simulink model "SwPenSUSim_US1"  (R2021a)
settings: Solver=ode14x  StartTime=0.0  StopTime=100  FixedStep=0.001  MaxStep=0.001  RelTol=1e5
undefined symbols (not defined in the file or in its folder): X, Y, Z
libraries: sm_lib x15, nesl_utility x3
settings Model: Creator=User  LastModifiedBy=sujay
settings SolverCC: SolverJacobianMethodControl=FullAnalytical  ZeroCrossControl=DisableAll  AlgebraicLoopSolver=TrustRegion  SolverResetMethod=Robust
settings DataIOCC: ReturnWorkspaceOutputs=off
settings DebuggingCC: SFMachineParentedDataDiag=warning  ArithmeticOperatorsInVariantConditions=warning
settings SFSimCC: SimUseLocalCustomCode=off  CustomCodeUndefinedFunction=UseInterfaceOnly
settings RTWCC: RTWUseLocalCustomCode=off
settings CodeAppCC: StateflowObjectComments=on
settings SimscapeCC: SimscapeNormalizeSystem=off
settings ExplorerConfigSet: InternalSimMechanicsExplorerSettings="<ExplorerConfiguration><canonicalview>default</canonicalview><AnimationSetting><BasePlaybackSpeed>1.0</BasePlaybackSpeed><PlaybackSpeedFactor>1.0</PlaybackSpeedFactor></AnimationSetting><TilePanel><TileInfo><Tiles Columns=\"2\" Count=\"4\" Rows=\"2\"><Column Weight=\"0.4995\"/><Column Weight=\"0.5005\"/><Row Weight=\"0.5\"/><Row Weight=\"0.5\"/><Tile Height=\"1\" Width=\"1\" X=\"0\" Y=\"0\"/><Tile Height=\"1\" Width=\"1\" X=\"0\" Y=\"1\"/><Tile Height=\"1\" Width=\"1\" X=\"1\" Y=\"0\"/><Tile Height=\"1\" Width=\"1\" X=\"1\" Y=\"1\"/></Tiles></TileInfo><SceneInfo><SceneViewer><BGColor><R>0.60000002384185791</R><G>0.60000002384185791</G><B>0.60000002384185791</B></BGColor><Camera><DoPerspective>off</DoPerspective><Position><X>-0.0531052448703034363</X><Y>-1</Y><Z>-0.0866656671353977226</Z></Position><Center><X>-0.0531052448703034363</X><Y>1.38777878078144568e-17</Y><Z>-0.0866656671353977226</Z></Center><Up><X>0</X><Y>-0</Y><Z>1</Z></Up><ViewLimDist>1</ViewLimDist><YLim>0.890956787716308041</YLim><XLim>1.8773732312593634</XLim></Camera></SceneViewer><SceneViewer><BGColor><R>0.60000002384185791</R><G>0.60000002384185791</G><B>0.60000002384185791</B></BGColor><Camera><DoPerspective>off</DoPerspective><Position><X>-0.0296964864584461918</X><Y>-0.0267970504804747045</Y><Z>0.876248933374882633</Z></Position><Center><X>-0.0296964864584461918</X><Y>-0.0267970504804747045</Y><Z>-0.123751066625117367</Z></Center><Up><X>0</X><Y>1</Y><Z>-0</Z></Up><ViewLimDist>1</ViewLimDist><YLim>0.835585083440608556</YLim><XLim>1.76069714010699663</XLim></Camera></SceneViewer><SceneViewer><BGColor><R>0.60000002384185791</R><G>0.60000002384185791</G><B>0.60000002384185791</B></BGColor><Camera><DoPerspective>off</DoPerspective><Position><X>1</X><Y>-0.0387358476867863816</Y><Z>-0.0757430226595436767</Z></Position><Center><X>0</X><Y>-0.0387358476867863816</Y><Z>-0.0757430226595436767</Z></Center><Up><X>-0</X><Y>0</Y><Z>1</Z></Up><ViewLimDist>1</ViewLimDist><YLim>0.674834154997757341</YLim><XLim>1.42347829569839446</XLim></Camera></SceneViewer><SceneViewer><BGColor><R>0.60000002384185791</R><G>0.60000002384185791</G><B>0.60000002384185791</B></BGColor><Camera><DoPerspective>off</DoPerspective><Position><X>0.534397979001275503</X><Y>-0.548841185035268575</Y><Z>0.55129295382820287</Z></Position><Center><X>-0.0429522901883504296</X><Y>0.0285090841543572567</Y><Z>-0.0260573153614229794</Z></Center><Up><X>-0.408248290463863073</X><Y>0.408248290463863073</Y><Z>0.816496580927726145</Z></Up><ViewLimDist>1</ViewLimDist><YLim>0.529378959523886694</YLim><XLim>1.11665874274569843</XLim></Camera></SceneViewer></SceneInfo></TilePanel><MechEditorPanel><Cameras/><GfxPanelCameraMap/><VideoCreator><PlaybackSpeedRatio>1</PlaybackSpeedRatio><FrameRate>60</FrameRate><VideoFormat>MPEG-4</VideoFormat><FrameSize>[1920 1080]</FrameSize></VideoCreator></MechEditorPanel></ExplorerConfiguration>"

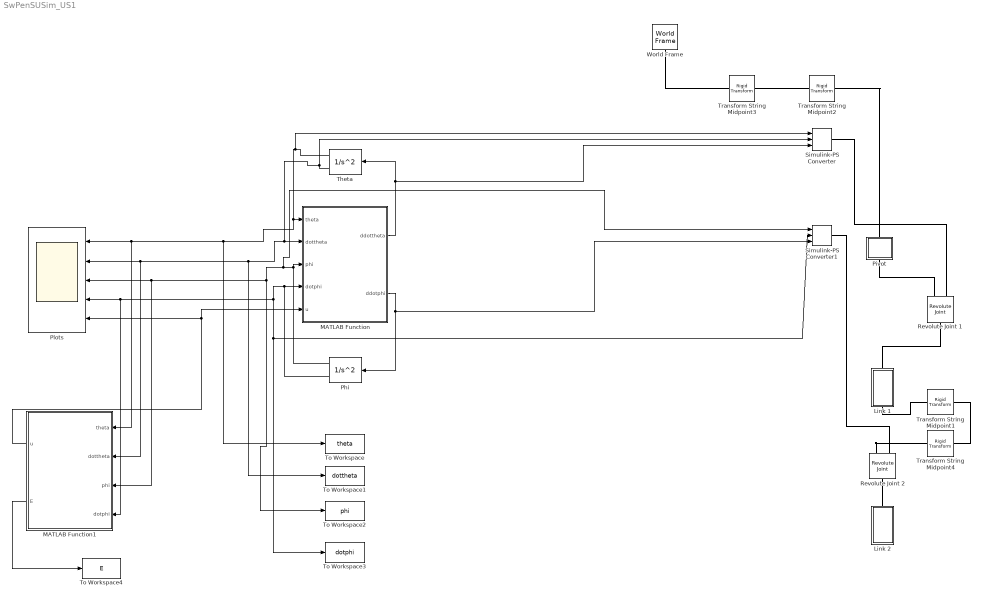
== system SwPenSUSim_US1 ==
  Link 1 : Subsystem  Tag=CustomStyle
  Link 2 : Subsystem  Tag=CustomStyle
  MATLAB Function : MATLAB Function  TreatAsAtomicUnit=on
  MATLAB Function1 : MATLAB Function  TreatAsAtomicUnit=on
  Phi : SecondOrderIntegrator  ICX=phi_0  UpperLimitX=2*pi  LowerLimitX=0  WrapX=on  ICDXDT=dphi_0  UpperLimitDXDT=15  LowerLimitDXDT=-15
  Pivot : Subsystem  Tag=CustomStyle
  Plots : Scope  NumInputPorts=5
  Revolute Joint 1 : sm_lib/Joints/Revolute Joint  JointMode=Normal  SenseConstraintForce=off  SenseConstraintForceX=off  SenseConstraintForceY=off  SenseConstraintForceZ=off  SenseConstraintTorque=off  SenseConstraintTorqueX=off  SenseConstraintTorqueY=off  SenseConstraintTorqueZ=off  SenseTotalForce=off  SenseTotalForceX=off  SenseTotalForceY=off  SenseTotalForceZ=off  SenseTotalTorque=off  SenseTotalTorqueX=off  SenseTotalTorqueY=off  SenseTotalTorqueZ=off  CompositeWrenchDir=FollowerOnBase  CompositeWrenchFrame=BaseFrame  EquilibriumPosition=0  EquilibriumPositionUnits=rad  SpringStiffness=0  SpringStiffnessUnits=N*m/rad  DampingCoefficient=0  DampingCoefficientUnits=N*m/(rad/s)  TorqueActuationMode=ComputedTorque  MotionActuationMode=InputMotion  SensePosition=off  SenseVelocity=off  SenseAcceleration=off  SenseTorqueForce=off  SenseLowerLimitTorqueForce=off  SenseUpperLimitTorqueForce=off  LowerLimitSpecify=off  LowerLimitBound=-90  LowerLimitBoundUnits=deg  LowerLimitStiffness=1e4  LowerLimitStiffnessUnits=N*m/deg  LowerLimitDamping=10  LowerLimitDampingUnits=N*m/(deg/s)  LowerLimitTransitionRegionWidth=0.1  LowerLimitTransitionRegionWidthUnits=deg  UpperLimitSpecify=off  UpperLimitBound=90  UpperLimitBoundUnits=deg  UpperLimitStiffness=1e4  UpperLimitStiffnessUnits=N*m/deg  UpperLimitDamping=10  UpperLimitDampingUnits=N*m/(deg/s)  UpperLimitTransitionRegionWidth=0.1  UpperLimitTransitionRegionWidthUnits=deg  PositionTargetSpecify=off  PositionTargetPriority=High  PositionTargetValue=0  PositionTargetValueUnits=deg  VelocityTargetSpecify=off  VelocityTargetPriority=High  VelocityTargetValue=0  VelocityTargetValueUnits=rad/s
  Revolute Joint 2 : sm_lib/Joints/Revolute Joint  JointMode=Normal  SenseConstraintForce=off  SenseConstraintForceX=off  SenseConstraintForceY=off  SenseConstraintForceZ=off  SenseConstraintTorque=off  SenseConstraintTorqueX=off  SenseConstraintTorqueY=off  SenseConstraintTorqueZ=off  SenseTotalForce=off  SenseTotalForceX=off  SenseTotalForceY=off  SenseTotalForceZ=off  SenseTotalTorque=off  SenseTotalTorqueX=off  SenseTotalTorqueY=off  SenseTotalTorqueZ=off  CompositeWrenchDir=FollowerOnBase  CompositeWrenchFrame=BaseFrame  EquilibriumPosition=0  EquilibriumPositionUnits=rad  SpringStiffness=0  SpringStiffnessUnits=N*m/rad  DampingCoefficient=0  DampingCoefficientUnits=N*m/(rad/s)  TorqueActuationMode=ComputedTorque  MotionActuationMode=InputMotion  SensePosition=off  SenseVelocity=off  SenseAcceleration=off  SenseTorqueForce=off  SenseLowerLimitTorqueForce=off  SenseUpperLimitTorqueForce=off  LowerLimitSpecify=off  LowerLimitBound=-90  LowerLimitBoundUnits=deg  LowerLimitStiffness=1e4  LowerLimitStiffnessUnits=N*m/deg  LowerLimitDamping=10  LowerLimitDampingUnits=N*m/(deg/s)  LowerLimitTransitionRegionWidth=0.1  LowerLimitTransitionRegionWidthUnits=deg  UpperLimitSpecify=off  UpperLimitBound=90  UpperLimitBoundUnits=deg  UpperLimitStiffness=1e4  UpperLimitStiffnessUnits=N*m/deg  UpperLimitDamping=10  UpperLimitDampingUnits=N*m/(deg/s)  UpperLimitTransitionRegionWidth=0.1  UpperLimitTransitionRegionWidthUnits=deg  PositionTargetSpecify=off  PositionTargetPriority=High  PositionTargetValue=0  PositionTargetValueUnits=deg  VelocityTargetSpecify=off  VelocityTargetPriority=High  VelocityTargetValue=0  VelocityTargetValueUnits=rad/s
  Simulink-PS Converter : nesl_utility/Simulink-PS Converter  PhysicalDomain=network_engine_domain  SubClassName=ps_input  LeftPortType=input  RightPortType=output  PseudoPeriodic=off  Frequencies=[]  NoiseDistribution=none  NoiseParameters=[]  Unit=rad  AffineConversion=on  FilteringAndDerivatives=provide  SimscapeFilterOrder=1  InputFilterTimeConstant=0.001  UdotUserProvided=2
      settings: SourceProductBaseCode=PW,SS
  Simulink-PS Converter1 : nesl_utility/Simulink-PS Converter  PhysicalDomain=network_engine_domain  SubClassName=ps_input  LeftPortType=input  RightPortType=output  PseudoPeriodic=off  Frequencies=[]  NoiseDistribution=none  NoiseParameters=[]  Unit=rad  AffineConversion=on  FilteringAndDerivatives=provide  SimscapeFilterOrder=1  InputFilterTimeConstant=0.001  UdotUserProvided=2
      settings: SourceProductBaseCode=PW,SS
  Theta : SecondOrderIntegrator  ICX=theta_0  ICDXDT=dtheta_0  UpperLimitDXDT=15  LowerLimitDXDT=-15
  To Workspace : ToWorkspace  VariableName=theta  SampleTime=-1
  To Workspace1 : ToWorkspace  VariableName=dottheta  SampleTime=-1
  To Workspace2 : ToWorkspace  VariableName=phi  SampleTime=-1
  To Workspace3 : ToWorkspace  VariableName=dotphi  SampleTime=-1
  To Workspace4 : ToWorkspace  VariableName=E  SampleTime=-1
  Transform String Midpoint1 : sm_lib/Frames and Transforms/Rigid Transform  TranslationMethod=None  TranslationStandardOffset=0  TranslationLengthUnit=m  TranslationStandardAxis=-Y  TranslationCartesianOffset=[0 0 0]  TranslationROffset=0  TranslationROffsetUnits=m  TranslationZOffset=0  TranslationZOffsetUnits=m  TranslationThetaOffset=0  TranslationThetaOffsetUnits=deg  RotationMethod=StandardAxis  RotationAngleUnits=deg  RotationStandardAxis=-X  RotationAngle=90  RotationArbitraryAxis=[0 0 1]  FollAlignAxisA=+X  BaseAlignAxisA=+Y  FollAlignAxisB=+Y  BaseAlignAxisB=+Z  RotationSequenceAxes=FollowerAxes  RotationSequence=XYX  RotationSequenceAngles=[0 0 0]  RotationSequenceAnglesUnits=deg  RotationMatrix=[1 0 0; 0 1 0; 0 0 1]
  Transform String Midpoint2 : sm_lib/Frames and Transforms/Rigid Transform  TranslationMethod=None  TranslationStandardOffset=0  TranslationLengthUnit=m  TranslationStandardAxis=-Y  TranslationCartesianOffset=[0 0 0]  TranslationROffset=0  TranslationROffsetUnits=m  TranslationZOffset=0  TranslationZOffsetUnits=m  TranslationThetaOffset=0  TranslationThetaOffsetUnits=deg  RotationMethod=StandardAxis  RotationAngleUnits=deg  RotationStandardAxis=+X  RotationAngle=90  RotationArbitraryAxis=[0 0 1]  FollAlignAxisA=+X  BaseAlignAxisA=+Y  FollAlignAxisB=+Y  BaseAlignAxisB=+Z  RotationSequenceAxes=FollowerAxes  RotationSequence=XYX  RotationSequenceAngles=[0 0 0]  RotationSequenceAnglesUnits=deg  RotationMatrix=[1 0 0; 0 1 0; 0 0 1]
  Transform String Midpoint3 : sm_lib/Frames and Transforms/Rigid Transform  TranslationMethod=None  TranslationStandardOffset=0  TranslationLengthUnit=m  TranslationStandardAxis=-Y  TranslationCartesianOffset=[0 0 0]  TranslationROffset=0  TranslationROffsetUnits=m  TranslationZOffset=0  TranslationZOffsetUnits=m  TranslationThetaOffset=0  TranslationThetaOffsetUnits=deg  RotationMethod=StandardAxis  RotationAngleUnits=deg  RotationStandardAxis=+Y  RotationAngle=180  RotationArbitraryAxis=[0 0 1]  FollAlignAxisA=+X  BaseAlignAxisA=+Y  FollAlignAxisB=+Y  BaseAlignAxisB=+Z  RotationSequenceAxes=FollowerAxes  RotationSequence=XYX  RotationSequenceAngles=[0 0 0]  RotationSequenceAnglesUnits=deg  RotationMatrix=[1 0 0; 0 1 0; 0 0 1]
  Transform String Midpoint4 : sm_lib/Frames and Transforms/Rigid Transform  TranslationMethod=None  TranslationStandardOffset=0.15/2  TranslationLengthUnit=m  TranslationStandardAxis=-Y  TranslationCartesianOffset=[0 0 0]  TranslationROffset=0  TranslationROffsetUnits=m  TranslationZOffset=0  TranslationZOffsetUnits=m  TranslationThetaOffset=0  TranslationThetaOffsetUnits=deg  RotationMethod=StandardAxis  RotationAngleUnits=deg  RotationStandardAxis=-X  RotationAngle=180  RotationArbitraryAxis=[0 0 1]  FollAlignAxisA=+X  BaseAlignAxisA=+Y  FollAlignAxisB=+Y  BaseAlignAxisB=+Z  RotationSequenceAxes=FollowerAxes  RotationSequence=XYX  RotationSequenceAngles=[0 0 0]  RotationSequenceAnglesUnits=deg  RotationMatrix=[1 0 0; 0 1 0; 0 0 1]
  World Frame : sm_lib/Frames and Transforms/World Frame
  wires:
  Theta/2 -> Simulink-PS Converter/2, To Workspace1/1, MATLAB Function1/2(dottheta), Plots/2, MATLAB Function/2(dottheta)
  Phi/2 -> To Workspace3/1, Simulink-PS Converter1/2, MATLAB Function1/4(dotphi), Plots/4, MATLAB Function/4(dotphi)
  MATLAB Function/1(ddottheta) -> Simulink-PS Converter/3, Theta/1
  MATLAB Function/2(ddotphi) -> Simulink-PS Converter1/3, Phi/1
  MATLAB Function1/1(u) -> MATLAB Function/5(u), Plots/5
  Phi/1 -> Simulink-PS Converter1/1, To Workspace2/1, MATLAB Function1/3(phi), Plots/3, MATLAB Function/3(phi)
  Theta/1 -> Simulink-PS Converter/1, To Workspace/1, MATLAB Function1/1(theta), Plots/1, MATLAB Function/1(theta)
  MATLAB Function1/2(E) -> To Workspace4/1
  connections:
  Revolute Joint 2/LConn2 -- Simulink-PS Converter1/RConn1
  Transform String Midpoint1/LConn1 -- Transform String Midpoint4/LConn1
  Simulink-PS Converter/RConn1 -- Revolute Joint 1/LConn2
  Link 2/RConn1 -- Revolute Joint 2/RConn1
  Link 1/RConn1 -- Revolute Joint 1/RConn1
  Pivot/RConn1 -- Revolute Joint 1/LConn1
  Link 1/LConn1 -- Transform String Midpoint1/RConn1
  Transform String Midpoint2/LConn1 -- Pivot/LConn1
  Transform String Midpoint3/LConn1 -- Transform String Midpoint2/RConn1
  World Frame/RConn1 -- Transform String Midpoint3/RConn1
  Transform String Midpoint4/RConn1 -- Revolute Joint 2/LConn1

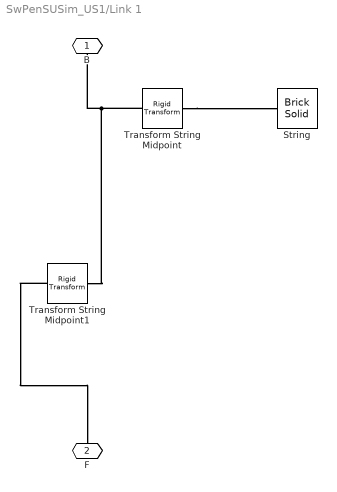
== system SwPenSUSim_US1/Link 1 ==
  String : sm_lib/Body Elements/Brick Solid  GraphicAmbientColor=[0.15 0.15 0.15 1.0]  BasedOnType=Density  BrickDimensions=[0.012 0.25 0.012]  BrickDimensionUnits=m  CenterOfMass=[0 0 0]  CenterOfMassUnits=m  GraphicDiffuseColor=[0.3764706 0.21568628 0.3764706]  Density=0  DensityUnits=kg/(m^3)  DoExposeReferenceFrame=on  GraphicEmissiveColor=[0.0 0.0 0.0 1.0]  ExportEntireGeometry=off  SerializedFrames=<Frames/>  MarkerShape=Sphere  MarkerSize=10  GraphicType=FromGeometry  InertiaType=PointMass  Mass=0  MassUnits=kg  MomentsOfInertia=[1 1 1]*1e-3  MomentsOfInertiaUnits=kg*m^2  GraphicOpacity=1.0  ProductsOfInertia=[0 0 0]  ProductsOfInertiaUnits=kg*m^2  GraphicShininess=75  GraphicSpecularColor=[0.5 0.5 0.5 1.0]  GraphicVisPropType=SimpleVisualProperties
  Transform String Midpoint : sm_lib/Frames and Transforms/Rigid Transform  TranslationMethod=StandardAxis  TranslationStandardOffset=0.25/2  TranslationLengthUnit=m  TranslationStandardAxis=-Y  TranslationCartesianOffset=[0 0 0]  TranslationROffset=0  TranslationROffsetUnits=m  TranslationZOffset=0  TranslationZOffsetUnits=m  TranslationThetaOffset=0  TranslationThetaOffsetUnits=deg  RotationMethod=None  RotationAngleUnits=deg  RotationStandardAxis=+Z  RotationAngle=0  RotationArbitraryAxis=[0 0 1]  FollAlignAxisA=+X  BaseAlignAxisA=+Y  FollAlignAxisB=+Y  BaseAlignAxisB=+Z  RotationSequenceAxes=FollowerAxes  RotationSequence=XYX  RotationSequenceAngles=[0 0 0]  RotationSequenceAnglesUnits=deg  RotationMatrix=[1 0 0; 0 1 0; 0 0 1]
  Transform String Midpoint1 : sm_lib/Frames and Transforms/Rigid Transform  TranslationMethod=StandardAxis  TranslationStandardOffset=0.25  TranslationLengthUnit=m  TranslationStandardAxis=-Y  TranslationCartesianOffset=[0 0 0]  TranslationROffset=0  TranslationROffsetUnits=m  TranslationZOffset=0  TranslationZOffsetUnits=m  TranslationThetaOffset=0  TranslationThetaOffsetUnits=deg  RotationMethod=None  RotationAngleUnits=deg  RotationStandardAxis=+Z  RotationAngle=0  RotationArbitraryAxis=[0 0 1]  FollAlignAxisA=+X  BaseAlignAxisA=+Y  FollAlignAxisB=+Y  BaseAlignAxisB=+Z  RotationSequenceAxes=FollowerAxes  RotationSequence=XYX  RotationSequenceAngles=[0 0 0]  RotationSequenceAnglesUnits=deg  RotationMatrix=[1 0 0; 0 1 0; 0 0 1]
  B : PMIOPort  Side=Right
  F : PMIOPort  Port=2  Side=Left
  connections:
  Transform String Midpoint/RConn1 -- String/RConn1
  Transform String Midpoint/LConn1 -- Transform String Midpoint1/LConn1 -- B/RConn1
  Transform String Midpoint1/RConn1 -- F/RConn1

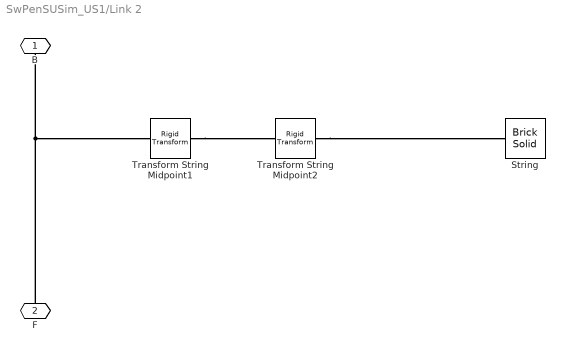
== system SwPenSUSim_US1/Link 2 ==
  String : sm_lib/Body Elements/Brick Solid  GraphicAmbientColor=[0.15 0.15 0.15 1.0]  BasedOnType=Density  BrickDimensions=[0.015 0.15 0.015]  BrickDimensionUnits=m  CenterOfMass=[0 0 0]  CenterOfMassUnits=m  GraphicDiffuseColor=[0.011764706 0.40392157 0.6392157]  Density=0  DensityUnits=kg/(m^3)  DoExposeReferenceFrame=on  GraphicEmissiveColor=[0.0 0.0 0.0 1.0]  ExportEntireGeometry=off  SerializedFrames=<Frames/>  MarkerShape=Sphere  MarkerSize=10  GraphicType=FromGeometry  InertiaType=PointMass  Mass=0  MassUnits=kg  MomentsOfInertia=[1 1 1]*1e-3  MomentsOfInertiaUnits=kg*m^2  GraphicOpacity=1.0  ProductsOfInertia=[0 0 0]  ProductsOfInertiaUnits=kg*m^2  GraphicShininess=75  GraphicSpecularColor=[0.5 0.5 0.5 1.0]  GraphicVisPropType=SimpleVisualProperties
  Transform String Midpoint1 : sm_lib/Frames and Transforms/Rigid Transform  TranslationMethod=StandardAxis  TranslationStandardOffset=0.15/2  TranslationLengthUnit=m  TranslationStandardAxis=-Y  TranslationCartesianOffset=[0 0 0]  TranslationROffset=0  TranslationROffsetUnits=m  TranslationZOffset=0  TranslationZOffsetUnits=m  TranslationThetaOffset=0  TranslationThetaOffsetUnits=deg  RotationMethod=StandardAxis  RotationAngleUnits=deg  RotationStandardAxis=-Z  RotationAngle=180  RotationArbitraryAxis=[0 0 1]  FollAlignAxisA=+X  BaseAlignAxisA=+Y  FollAlignAxisB=+Y  BaseAlignAxisB=+Z  RotationSequenceAxes=FollowerAxes  RotationSequence=XYX  RotationSequenceAngles=[0 0 0]  RotationSequenceAnglesUnits=deg  RotationMatrix=[1 0 0; 0 1 0; 0 0 1]
  Transform String Midpoint2 : sm_lib/Frames and Transforms/Rigid Transform  TranslationMethod=None  TranslationStandardOffset=0.15/2  TranslationLengthUnit=m  TranslationStandardAxis=-Y  TranslationCartesianOffset=[0 0 0]  TranslationROffset=0  TranslationROffsetUnits=m  TranslationZOffset=0  TranslationZOffsetUnits=m  TranslationThetaOffset=0  TranslationThetaOffsetUnits=deg  RotationMethod=StandardAxis  RotationAngleUnits=deg  RotationStandardAxis=+X  RotationAngle=0  RotationArbitraryAxis=[0 0 1]  FollAlignAxisA=+X  BaseAlignAxisA=+Y  FollAlignAxisB=+Y  BaseAlignAxisB=+Z  RotationSequenceAxes=FollowerAxes  RotationSequence=XYX  RotationSequenceAngles=[0 0 0]  RotationSequenceAnglesUnits=deg  RotationMatrix=[1 0 0; 0 1 0; 0 0 1]
  B : PMIOPort  Side=Right
  F : PMIOPort  Port=2  Side=Left
  connections:
  Transform String Midpoint1/LConn1 -- Transform String Midpoint2/RConn1
  F/RConn1 -- Transform String Midpoint1/RConn1 -- B/RConn1
  Transform String Midpoint2/LConn1 -- String/RConn1

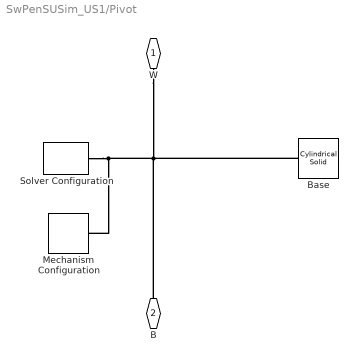
== system SwPenSUSim_US1/Pivot ==
  Base : sm_lib/Body Elements/Cylindrical Solid  GraphicAmbientColor=[0.15 0.15 0.15 1.0]  BasedOnType=Density  CenterOfMass=[0 0 0]  CenterOfMassUnits=m  GraphicDiffuseColor=[0.3 0.3 0.3]  CylinderLength=0.4  CylinderLengthUnits=m  CylinderRadius=0.01  CylinderRadiusUnits=m  Density=1000  DensityUnits=kg/(m^3)  DoExposeReferenceFrame=on  GraphicEmissiveColor=[0.0 0.0 0.0 1.0]  ExportEntireGeometry=off  SerializedFrames=<Frames/>  MarkerShape=Sphere  MarkerSize=10  GraphicType=FromGeometry  InertiaType=PointMass  Mass=10  MassUnits=kg  MomentsOfInertia=[1 1 1]*1e-3  MomentsOfInertiaUnits=kg*m^2  GraphicOpacity=1.0  ProductsOfInertia=[0 0 0]  ProductsOfInertiaUnits=kg*m^2  GraphicShininess=75  GraphicSpecularColor=[0.5 0.5 0.5 1.0]  GraphicVisPropType=AdvancedVisualProperties
  Mechanism Configuration : sm_lib/Utilities/Mechanism Configuration  UniformGravity=Constant  GravityVector=[0 0 -9.81]  GravityVectorUnits=m/s^2  GravityUnits=m/s^2  LinearizationDelta=0.001  JointModeTransitionNonlinearIterations=2
  Solver Configuration : nesl_utility/Solver Configuration  PhysicalDomain=network_engine_domain  SubClassName=solver  LeftPortType=input  RightPortType=generic  Tones=[]  Harmonics=[]  SimulateNoise=off  Profile=off  UseLocalSampling=off  EnableSwitchedLinearOptims=on  FrequencyDomain=off  UseCCode=off  RelTol=0.001  AbsTol=1e-06  MinStep=1e-09  ToWorkspace=off  RevertToSquareIcSolve=off  NumHomotopyIterations=100  PhasorMode=off  PhasorModeNumHarmonics=1  DoDC=on  ResidualTolerance=1e-9  UseLocalSolver=off  LocalSolverChoice=NE_BACKWARD_EULER_ADVANCER  LocalSolverSampleTime=.001  DoFixedCost=off  MaxNonlinIter=3  MaxModeIter=2  ComputeImpulses=off  ImpulseIterations=2  LinearAlgebra=Sparse  EquationFormulation=NE_TIME_EF  DelaysMemoryBudget=1024  AutomaticFiltering=on  FilteringTimeConstant=0.001  PartitionStorageMethod=AS_NEEDED  PartitionMemoryBudget=1024  PartitionMethod=FAST
      settings: SourceProductBaseCode=PW,SS
  W : PMIOPort  Side=Left
  B : PMIOPort  Port=2  Side=Right
  connections:
  W/RConn1 -- B/RConn1 -- Base/RConn1 -- Solver Configuration/RConn1 -- Mechanism Configuration/RConn1

== matlab function SwPenSUSim_US1/MATLAB Function1 ==
  data: theta input; dottheta input; phi input; dotphi input; u output; E output
function [u,E] =SwirlingPendulum(theta,dottheta,phi,dotphi)
%% Swirling Pendulum Equations of Motion
% Define the parameter values
% u=0;
m1 = 0.435;
m2 = 0.325;
l1 = 0.07;
l2 = 0.0855;
g = 9.81;
% % Inertia Matrix
M=[4/3*(m1*l1^2+m2*(3*l1^2+(l2*sin(phi))^2)), 2*m2*l1*l2*cos(phi);
    2*m2*l1*l2*cos(phi), 4/3*(m2*l2^2)];
% Coriolis 
C=[0 8/3*(m2*l2^2)*sin(phi)*cos(phi)*dottheta-2*m2*l1*l2*sin(phi)*dotphi;-4/3*m2*l2^2*cos(phi)*sin(phi)*dottheta 0];
% Potential Terms
G=[(m1+2*m2)*g*l1*sin(theta)+m2*g*l2*sin(phi)*cos(theta);
    m2*g*l2*sin(theta)*cos(phi)];
B=[0;1];
x=[theta;phi;dottheta;dotphi];
% F1=[dottheta;dotphi];
% f1=F1(1,:);
% f2=F1(2,:);
% F2=pinv(M)*(-C*[dottheta;dotphi]-G);
% f3=F2(1,:);
% f4=F2(2,:);
% G1=[0;0];
% G2=pinv(M)*B;
% g1=G1(1,:);
% g2=G1(2,:);
% g3=G2(1,:);
% g4=G2(2,:);
% xdot=[f1;f2;f3;f4]+[g1;g2;g3;g4]*u;
E=((1/2*([dottheta;dotphi]'*M*[dottheta;dotphi])+m2*g*l2*sin(phi)*sin(theta)-2*m2*g*l1*cos(theta)-m1*g*l1*cos(theta)));
% K=1*[-9.0033 0.6258 0.0239 0.5591];
% K=[-2.8177    0.2843   -0.0085    0.1793]
% K=[-0.5894    0.1781   -0.0118    0.0480];
% K=[-6.3550    0.4784    0.0095    0.3962]; % Works well
% K=[-20.1762    1.2513    0.0852    1.2475];
% K=[-63.8740    3.7026    0.3268    3.9411];
% K=[-202.0556   11.4565    1.0914   12.4594];
% K=[-285.7627   16.1538    1.5546   17.6196];
% K=[-286.0944   16.0296    0.2667  101.0471];
% K=[-262.6306  -72.9283  -12.6208   20.7545];
% K=[-283.1572  -62.3050  -11.4901   21.2444];
% S=K*x;
% ksw=0.00001;
% u_sw=0;
% u_eq=0;
% u=0;
% u_sw=-ksw*S*sign(S);
% u_eq=-pinv(K*[0;0;-270.6055;626.1394])*(K*[0 0 1 0;0 0 0 1;-92.5253 -62.9094 0 0;26.9446 75.4913 0 0]*[theta;phi;dottheta;dotphi]);
% u=u_eq+u_sw;
% u=-tanh(dotphi)*dotphi;
%%
% mu=[0 1]*pinv(M)*[0;1];
% K=0.001*[1 1];
% Kphi=1;
% Kphidot=1;
% Ke=1;
% u=dotphi*(K/(Kphi*mu)*(pinv(M)*(G+C*[dottheta;dotphi]-Ke*(E)-Kphidot*phi)));
%%
% mu=[0 1]*pinv(M)*[0;1];
% K=-0.25;
% Kphi=0.1;
% Kphidot=10;
% Ke=-0.01*0;
% kdel=1;
% kw=1;
% kphi=Kphi;
% ke=Ke;
% if (abs(phi)>pi/2-0.25) || (abs(dotphi)>2)
%     K=1;
% Kphi=1000000;
% Kphidot=0.1;
% Ke=0.1;
% end
% if (abs(theta)>0.5)
%     K=1;
% Kphi=1000000;
% Kphidot=0.1;
% Ke=0.1;
% end
% KK=0.0*[-16.0056 -6.4427 -0.2425 -0.1864];
%%
% u=1/(Kphi*mu)*(Kphi*[0 1]*pinv(M)*(G+C*[dottheta;dotphi])-Kphidot*(phi)+K*dotphi-Ke*(E));
% if abs(pi-theta)<0.1
%     u=-KK*(x+[-pi;0;0;0]);
% end
%%
% u=-(dottheta+dotphi+f3+f4)/(g3+g4)-0.001*sign(phi-pi/2);
% u=-(dottheta+dotphi+f3+f4)/(g3+g4)-0.001*tanh(phi-0*pi/2);
% KK=1*[-25.8922   -7.3486   -1.2980    2.0620];
% S=KK*x;
% usw=-0.3*tanh(S);
% % u=-(dottheta+dotphi+f3+f4)/(g3+g4)-0.001*tanh(phi-0*pi/2)-0.001*tanh(theta-0*pi/2);
% u=-(dottheta+dotphi+f3+f4)/(g3+g4)+usw;
%%
% if E<0.8
%     u = -(kdel*dotphi + kphi*dotphi*phi + (9*l1*cos(phi)*(dotphi*((8*m2*cos(phi)*sin(phi)*dottheta*l2^2)/3 - 2*l1*m2*sin(phi)*dotphi*l2) + g*l1*sin(theta)*(m1 + 2*m2) + g*l2*m2*cos(theta)*sin(phi)))/(8*l1^2*l2*m1 + 24*l1^2*l2*m2 + 8*l2^3*m2*sin(phi)^2 - 18*l1^2*l2*m2*cos(phi)^2) - (kw*dotphi*(3*g*l2*m2*cos(phi)*sin(theta) - 8*l2^2*m2*cos(phi)*sin(phi)*dottheta^2)*(l1^2*m1 + 3*l1^2*m2 + l2^2*m2*sin(phi)^2))/(12*l1^2*l2^2*m2^2 - 9*l1^2*l2^2*m2^2*cos(phi)^2 + 4*m1*l1^2*l2^2*m2 + 4*l2^4*m2^2*sin(phi)^2))/(ke*dotphi*(dottheta*((dottheta*((4*m2*(3*l1^2 + l2^2*sin(phi)^2))/3 + (4*l1^2*m1)/3))/2 + l1*l2*m2*cos(phi)*dotphi) + dotphi*((2*m2*dotphi*l2^2)/3 + l1*m2*cos(phi)*dottheta*l2) - g*l1*cos(theta)*(m1 + 2*m2) + g*l2*m2*sin(phi)*sin(theta)) + (3*kw*dotphi*(l1^2*m1 + 3*l1^2*m2 + l2^2*m2*sin(phi)^2))/(12*l1^2*l2^2*m2^2 - 9*l1^2*l2^2*m2^2*cos(phi)^2 + 4*m1*l1^2*l2^2*m2 + 4*l2^4*m2^2*sin(phi)^2)) ;
% end

%%
Ed=-0.7450695;
% Ed=0.75;
% k0=250;k1=0.5;k2=0.6;k3=2;
% k0=200;k1=0.5;k2=0.6;k3=2;
% k0=10000;k1=10;k2=1;k3=1;
% Ud=k2*g4+k0*(E-Ed);
% if abs(k2*g4+k0*(E-Ed))<0.01
%    Ud=0.01; 
% end
% if E>(-0.5)
%     k0=150;k1=1;k2=0.99;k3=2;
% end
% if E>0.5
%     k0=500;k1=1;k2=0.99;k3=2;
% end
% if E>0.5
%     k0=1000;k1=1;k2=1;k3=2;
% end
% if E>0.5
%     k0=250;k1=3;k2=1;k3=2;
% end
% if E<0.74
% u=-1*[-8.2967   -3.2349   -0.9178   -0.3590]*[(theta-pi);phi;dottheta;dotphi];
% u=-[-15.0777   -5.6164   -1.5838   -0.6078]*[(theta-pi);phi;dottheta;dotphi];
u=-0.1*tanh([-8.1253   -3.0735   -0.8961   -0.3386]*[(theta-pi);phi;dottheta;dotphi]);
%     if (abs(theta))>1
%         u=-1*(k1*phi+k2*f4+k3*dotphi)/Ud;
%     end
% end
% if (E<=Ed-0.001)&&(E>0.74)&&(abs(theta)>3.05)&&(abs(theta)<pi-0.0001)
%     KK=1*[-2.5469   -1.0316   -0.1675   -0.0614];
% S=-KK*[-(theta-pi);phi;dottheta;dotphi];
% usw=-0.3*tanh(S);
% u=-1*(k1*phi+k2*f4+k3*dotphi)/Ud+usw;
% end

% if (abs(theta)>3)
%     u=-0.001*[-66.9434  0   0   0]*[sign(theta)*abs(theta-pi);phi;dottheta;dotphi];
% end
% if (abs(theta)>3.1)
%     u=-1*[-23.7583   -8.9026   -2.6375   -1.0376]*[-sin(theta-pi);phi;dottheta;dotphi];
% end
% if (abs(theta)>3.05)&&(abs(theta)<pi-0.0001)
%     u=-1.0*[-0*2.5469   -0*1.0316   -0.1675   -0.0614]*[-(theta-pi);phi;dottheta;dotphi];
% end

== matlab function SwPenSUSim_US1/MATLAB Function ==
  data: theta input; dottheta input; phi input; dotphi input; u input; ddottheta output; ddotphi output
function [ddottheta,ddotphi]=SwirlingPendulum(theta,dottheta,phi,dotphi,u)
%% Swirling Pendulum Equations of Motion
% Define the parameter values
m1 = 0.435;
m2 = 0.325;
l1 = 0.07;
l2 = 0.0855;
g = 9.81;
% Inertia Matrix
M=[4/3*(m1*l1^2+m2*(3*l1^2+(l2*sin(phi))^2)), 2*m2*l1*l2*cos(phi);
    2*m2*l1*l2*cos(phi), 4/3*(m2*l2^2)];
% Coriolis 
C=[0 8/3*(m2*l2^2)*sin(phi)*cos(phi)*dottheta-2*m2*l1*l2*sin(phi)*dotphi;-4/3*m2*l2^2*cos(phi)*sin(phi)*dottheta 0];
% Potential Terms
G=[(m1+2*m2)*g*l1*sin(theta)+m2*g*l2*sin(phi)*cos(theta);
    m2*g*l2*sin(theta)*cos(phi)];
B=[0;1];
%Mx''+Cx'+G=Bu;
ddotX=inv(M)*(-C*[dottheta;dotphi]-G+B*u);
ddottheta=ddotX(1,:);
ddotphi=ddotX(2,:);
